simulink model "model_2"  (R2021b)
settings: Solver=ode23t  StartTime=0.0  StopTime=1e6
values from neighbouring files (symbols this model uses):
  Force_Vectors = [Force_Vectors;normal_vector]    [ellip_force_test.m]    (also in initial_sim.m = Force_Vectors'; initial_sim2.m = Force_Vectors'; multi_sim.m = Force_Vectors'; multi_sim2.m = Force_Vectors')
  max_f = 100000    [initial_sim.m]    (also in initial_sim2.m = 10)
  max_M_available = max_M_available*0.7    [initial_sim.m]    (also in initial_sim2.m; multi_sim.m; multi_sim2.m)
  Moment_Vectors = [Moment_Vectors;cross([x y z],normal_vector)]    [ellip_force_test.m]    (also in initial_sim.m = Moment_Vectors'; initial_sim2.m = Moment_Vectors'; multi_sim.m = Moment_Vectors'; multi_sim2.m = Moment_Vectors')
  N_sat = length(azimuths)    [ellip_force_test.m]    (also in initial_sim.m = 30; initial_sim2.m = 25; multi_sim.m = sim_data.N_sat; multi_sim2.m = sim_data.N_sat)
  params = 0    [Combo_OT.m]
undefined symbols (not defined in the file or in its folder): mp_0, mp_f
libraries: slpidlib x3, simulink x2, shared6dof x1
settings Model: Creator=Mehdi  LastModifiedBy=Mehdi

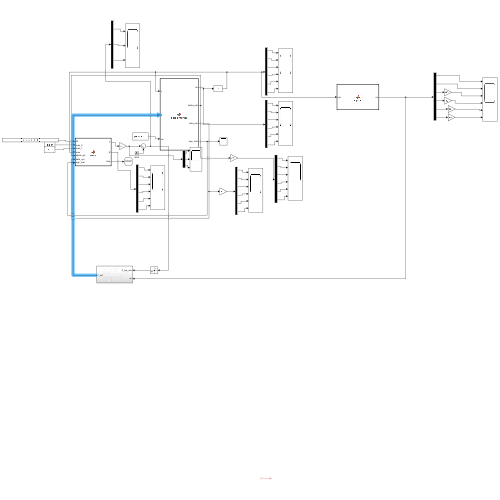
[thumbnail: Simulink's stored preview of the top-level diagram]
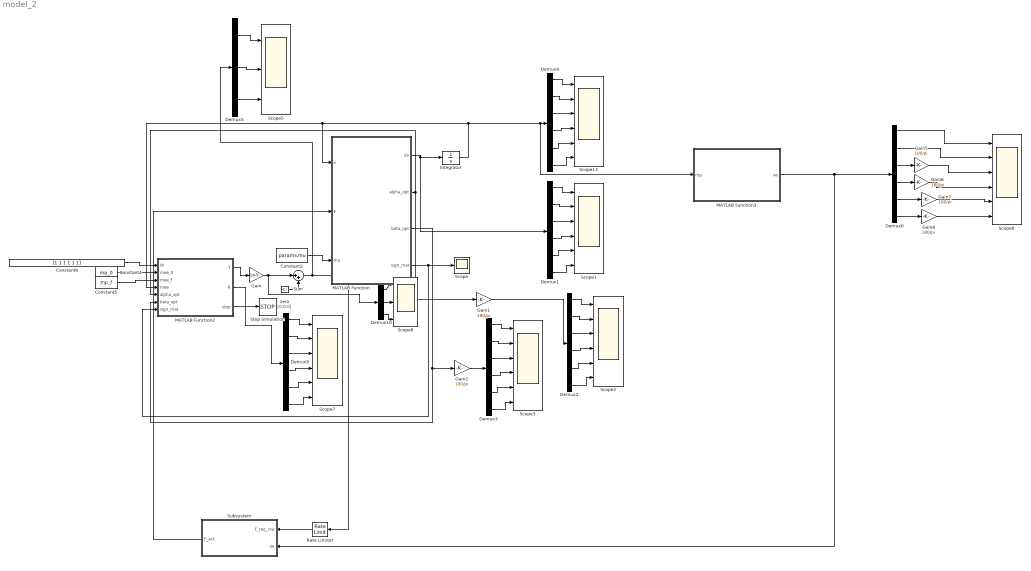
== system model_2 ==
  Constant2 : Constant  Value=params.mu
  Constant4 : Constant  Value=mp_0
  Constant5 : Constant  Value=mp_f
  Constant6 : Constant  Value=[1 1 1 1 1 1]
  Demux{1..3,6,8..9} (6 alike) : Demux  Outputs=6
  Demux10 : Demux  Outputs=3
  Demux5 : Demux  Outputs=3
  Gain : Gain  Gain=1e-5
  Gain{1..2,5..8} (6 alike) : Gain  Gain=180/pi
  Integrator : Integrator  InitialCondition=mp_0
  MATLAB Function : MATLAB Function  TreatAsAtomicUnit=on
  MATLAB Function2 : MATLAB Function  TreatAsAtomicUnit=on
  MATLAB Function3 : MATLAB Function  TreatAsAtomicUnit=on
  Rate Limiter : RateLimiter  RisingSlewLimit=1e-5  FallingSlewLimit=-1e-5  SampleTimeMode=inherited
  Scope : Scope
  Scope{1..3,6..7,13} (6 alike) : Scope  NumInputPorts=6
  Scope5 : Scope  NumInputPorts=3
  Scope8 : Scope  NumInputPorts=3
  Stop Simulation : Stop
  Subsystem : Subsystem
  Sum : Sum  Inputs=|++
  zero : Constant  Value=[0;0;0]
  wires:
  Integrator/1 -> MATLAB Function2/4(mee), MATLAB Function/1(x), MATLAB Function3/1(mp), Demux9/1
  Constant2/1 -> MATLAB Function/3(mu)
  Demux9/5 -> Scope13/5
  Demux9/1 -> Scope13/1
  Demux9/4 -> Scope13/4
  Demux9/3 -> Scope13/3
  Demux9/2 -> Scope13/2
  Demux9/6 -> Scope13/6
  Demux1/6 -> Scope1/6
  Demux1/2 -> Scope1/2
  Demux1/3 -> Scope1/3
  Demux1/4 -> Scope1/4
  Demux1/1 -> Scope1/1
  Demux1/5 -> Scope1/5
  Demux2/6 -> Scope2/6
  Demux2/2 -> Scope2/2
  Demux2/3 -> Scope2/3
  Demux2/4 -> Scope2/4
  Demux2/1 -> Scope2/1
  Demux2/5 -> Scope2/5
  MATLAB Function/2(alpha_opt) -> Gain1/1, MATLAB Function2/5(alpha_opt)
  MATLAB Function/3(beta_opt) -> MATLAB Function2/6(beta_opt), Gain2/1
  Demux3/5 -> Scope3/5
  Demux3/1 -> Scope3/1
  Demux3/4 -> Scope3/4
  Demux3/3 -> Scope3/3
  Demux3/2 -> Scope3/2
  Demux3/6 -> Scope3/6
  Constant4/1 -> MATLAB Function2/2(mee_0)
  Constant5/1 -> MATLAB Function2/3(mee_f)
  Constant6/1 -> MATLAB Function2/1(W)
  Demux5/3 -> Scope5/3
  Demux5/2 -> Scope5/2
  Demux5/1 -> Scope5/1
  MATLAB Function2/1(T) -> Gain/1
  zero/1 -> Sum/2
  Gain/1 -> Sum/1, Demux10/1
  MATLAB Function2/3(stop) -> Stop Simulation/1
  Demux6/6 -> Gain8/1
  Demux6/3 -> Gain5/1
  Demux6/4 -> Gain6/1
  Demux6/5 -> Gain7/1
  MATLAB Function3/1(oe) -> Subsystem/2(oe), Demux6/1
  Demux8/4 -> Scope7/4
  Demux8/3 -> Scope7/3
  Demux8/5 -> Scope7/5
  Demux8/2 -> Scope7/2
  Demux8/6 -> Scope7/6
  Demux8/1 -> Scope7/1
  MATLAB Function2/2(R) -> Demux8/1
  Gain1/1 -> Demux2/1
  MATLAB Function/1(dx) -> Demux1/1, Integrator/1
  Gain2/1 -> Demux3/1
  Demux6/1 -> Scope6/1
  Demux6/2 -> Scope6/2
  Gain5/1 -> Scope6/3
  Gain6/1 -> Scope6/4
  Gain7/1 -> Scope6/5
  Gain8/1 -> Scope6/6
  Demux10/2 -> Scope8/2
  Demux10/1 -> Scope8/1
  Demux10/3 -> Scope8/3
  ? -> ?
  Sum/1 -> Demux5/1, Rate Limiter/1
  Subsystem/1(F_act) -> MATLAB Function/2(F)
  Rate Limiter/1 -> Subsystem/1(F_req_rsw)
  MATLAB Function/4(sign_mat) -> MATLAB Function2/7(sign_mat), Scope/1

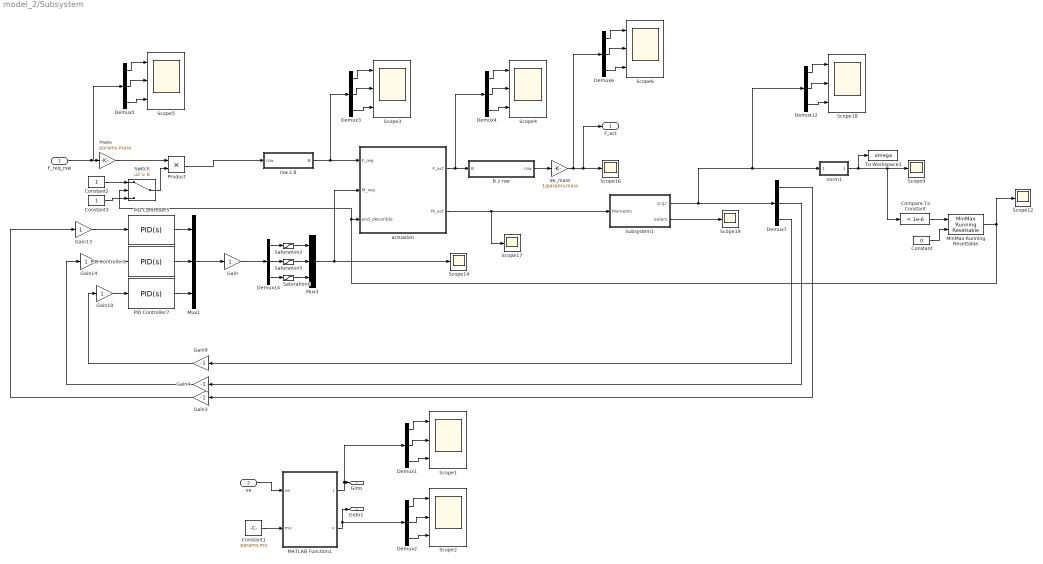
== system model_2/Subsystem ==
  F_req_rsw : Inport
  oe : Inport  Port=2
  B 2 rsw : Subsystem
  Compare To Constant : simulink/Logic and Bit Operations/Compare To Constant  relop=<  const=1e-6  OutDataTypeStr=boolean
  Constant : Constant  Value=0
  Constant1 : Constant  Value=params.mu
  Constant2 : Constant
  Constant3 : Constant
  Demux{1..7,12,14} (9 alike) : Demux  Outputs=3
  Gain{,10,13..14} (4 alike) : Gain
  Gain3 : Gain  Gain=-1
  Gain4 : Gain  Gain=-1
  Gain9 : Gain  Gain=-1
  MATLAB Function1 : MATLAB Function  TreatAsAtomicUnit=on
  MinMax Running Resettable : simulink/Math Operations/MinMax Running Resettable  Function=max  vinit=0.0
  Mux1 : Mux  Inputs=3
  Mux3 : Mux  Inputs=3
  PID Controller5 : slpidlib/PID Controller  Controller=PID  Form=Parallel  TimeDomain=Continuous-time  UseExternalTs=off  SampleTime=-1  IntegratorMethod=Forward Euler  FilterMethod=Forward Euler  ControllerParametersSource=internal  P=493.267124009933  I=0.0943532881280952  D=-103949.358808414  UseFilter=on  N=0.00172044274974478  TunerSelectOption=Transfer Function Based (PID Tuner App)  InitialConditionSource=internal  InitialConditionForIntegrator=0  InitialConditionForFilter=0  DifferentiatorICPrevScaledInput=0  ExternalReset=none  TrackingMode=off  Kt=1  LimitOutput=off  SatLimitsSource=internal  UpperSaturationLimit=inf  LowerSaturationLimit=-inf  LinearizeAsGain=on  AntiWindupMode=none  Kb=1  POutMin=[]  POutMax=[]  IOutMin=[]  IOutMax=[]  DOutMin=[]  DOutMax=[]  NOutMin=[]  NOutMax=[]  SumOutMin=[]  SumOutMax=[]  SaturationOutMin=[]  SaturationOutMax=[]  PParamMin=[]  PParamMax=[]  IParamMin=[]  IParamMax=[]  DParamMin=[]  DParamMax=[]  NParamMin=[]  NParamMax=[]  KbParamMin=[]  KbParamMax=[]  KtParamMin=[]  KtParamMax=[]  KbOutMin=[]  KbOutMax=[]  KtOutMin=[]  KtOutMax=[]  IntegratorOutMin=[]  IntegratorOutMax=[]  FilterOutMin=[]  FilterOutMax=[]  SumI1OutMin=[]  SumI1OutMax=[]  SumI2OutMin=[]  SumI2OutMax=[]  SumI3OutMin=[]  SumI3OutMax=[]  SumI4OutMin=[]  SumI4OutMax=[]  SumDOutMin=[]  SumDOutMax=[]  DifferentiatorOutMin=[]  DifferentiatorOutMax=[]  FilterDiffOutCoefMin=[]  FilterDiffOutCoefMax=[]  ReciprocalOutMin=[]  ReciprocalOutMax=[]  SumDenOutMin=[]  SumDenOutMax=[]  SumNumOutMin=[]  SumNumOutMax=[]  DivideOutMin=[]  DivideOutMax=[]  UdiffTsProdOutMin=[]  UdiffTsProdOutMax=[]  NTsProdOutMin=[]  NTsProdOutMax=[]  UintegralTsProdOutMin=[]  UintegralTsProdOutMax=[]  UngainTsProdOutMin=[]  UngainTsProdOutMax=[]  IntegratorContinuousStateAttributes=''  IntegratorStateMustResolveToSignalObject=off  IntegratorRTWStateStorageClass=Auto  FilterContinuousStateAttributes=''  FilterStateMustResolveToSignalObject=off  FilterRTWStateStorageClass=Auto  ParallelPVariant=InternalParameters  IdealPVariant=Disabled  IVariant=InternalParameters  DVariant=InternalParameters  IntegratorVariant=Continuous  SatVariant=Disabled  AWVariant=Passthrough  PCopyVariant=Disabled  TRVariant=Disabled  FdbkBlocksVariant=Forward  IdealPFdbkVariant=Disabled  SatFdbkVariant=Disabled  DerivativeFilterVariant=ContFilter  NVariant=InternalParameters  NCopyVariant=Disabled  FilterICVariant=InternalICsFilter  IntegratorICVariant=InternalICs  ExternalResetVariant=Disabled  TRSumVariant=Passthrough  SumFdbkVariant=Disabled  SumVariant=Sum_PID  TsampFilterVariant=InternalTs  TsampNgainVariant=Passthrough  TsampIntegralVariant=Passthrough  ExternalSaturationOutDataTypeStr=Inherit: Same as second input
  PID Controller6 : slpidlib/PID Controller  Controller=PID  Form=Parallel  TimeDomain=Continuous-time  UseExternalTs=off  SampleTime=-1  IntegratorMethod=Forward Euler  FilterMethod=Forward Euler  ControllerParametersSource=internal  P=493.267124009933  I=0.0943532881280952  D=-103949.358808414  UseFilter=on  N=0.00172044274974478  TunerSelectOption=Transfer Function Based (PID Tuner App)  InitialConditionSource=internal  InitialConditionForIntegrator=0  InitialConditionForFilter=0  DifferentiatorICPrevScaledInput=0  ExternalReset=none  TrackingMode=off  Kt=1  LimitOutput=off  SatLimitsSource=internal  UpperSaturationLimit=inf  LowerSaturationLimit=-inf  LinearizeAsGain=on  AntiWindupMode=none  Kb=1  POutMin=[]  POutMax=[]  IOutMin=[]  IOutMax=[]  DOutMin=[]  DOutMax=[]  NOutMin=[]  NOutMax=[]  SumOutMin=[]  SumOutMax=[]  SaturationOutMin=[]  SaturationOutMax=[]  PParamMin=[]  PParamMax=[]  IParamMin=[]  IParamMax=[]  DParamMin=[]  DParamMax=[]  NParamMin=[]  NParamMax=[]  KbParamMin=[]  KbParamMax=[]  KtParamMin=[]  KtParamMax=[]  KbOutMin=[]  KbOutMax=[]  KtOutMin=[]  KtOutMax=[]  IntegratorOutMin=[]  IntegratorOutMax=[]  FilterOutMin=[]  FilterOutMax=[]  SumI1OutMin=[]  SumI1OutMax=[]  SumI2OutMin=[]  SumI2OutMax=[]  SumI3OutMin=[]  SumI3OutMax=[]  SumI4OutMin=[]  SumI4OutMax=[]  SumDOutMin=[]  SumDOutMax=[]  DifferentiatorOutMin=[]  DifferentiatorOutMax=[]  FilterDiffOutCoefMin=[]  FilterDiffOutCoefMax=[]  ReciprocalOutMin=[]  ReciprocalOutMax=[]  SumDenOutMin=[]  SumDenOutMax=[]  SumNumOutMin=[]  SumNumOutMax=[]  DivideOutMin=[]  DivideOutMax=[]  UdiffTsProdOutMin=[]  UdiffTsProdOutMax=[]  NTsProdOutMin=[]  NTsProdOutMax=[]  UintegralTsProdOutMin=[]  UintegralTsProdOutMax=[]  UngainTsProdOutMin=[]  UngainTsProdOutMax=[]  IntegratorContinuousStateAttributes=''  IntegratorStateMustResolveToSignalObject=off  IntegratorRTWStateStorageClass=Auto  FilterContinuousStateAttributes=''  FilterStateMustResolveToSignalObject=off  FilterRTWStateStorageClass=Auto  ParallelPVariant=InternalParameters  IdealPVariant=Disabled  IVariant=InternalParameters  DVariant=InternalParameters  IntegratorVariant=Continuous  SatVariant=Disabled  AWVariant=Passthrough  PCopyVariant=Disabled  TRVariant=Disabled  FdbkBlocksVariant=Forward  IdealPFdbkVariant=Disabled  SatFdbkVariant=Disabled  DerivativeFilterVariant=ContFilter  NVariant=InternalParameters  NCopyVariant=Disabled  FilterICVariant=InternalICsFilter  IntegratorICVariant=InternalICs  ExternalResetVariant=Disabled  TRSumVariant=Passthrough  SumFdbkVariant=Disabled  SumVariant=Sum_PID  TsampFilterVariant=InternalTs  TsampNgainVariant=Passthrough  TsampIntegralVariant=Passthrough  ExternalSaturationOutDataTypeStr=Inherit: Same as second input
  PID Controller7 : slpidlib/PID Controller  Controller=PID  Form=Parallel  TimeDomain=Continuous-time  UseExternalTs=off  SampleTime=-1  IntegratorMethod=Forward Euler  FilterMethod=Forward Euler  ControllerParametersSource=internal  P=493.267124009933  I=0.0943532881280952  D=-103949.358808414  UseFilter=on  N=0.00172044274974478  TunerSelectOption=Transfer Function Based (PID Tuner App)  InitialConditionSource=internal  InitialConditionForIntegrator=0  InitialConditionForFilter=0  DifferentiatorICPrevScaledInput=0  ExternalReset=none  TrackingMode=off  Kt=1  LimitOutput=off  SatLimitsSource=internal  UpperSaturationLimit=inf  LowerSaturationLimit=-inf  LinearizeAsGain=on  AntiWindupMode=none  Kb=1  POutMin=[]  POutMax=[]  IOutMin=[]  IOutMax=[]  DOutMin=[]  DOutMax=[]  NOutMin=[]  NOutMax=[]  SumOutMin=[]  SumOutMax=[]  SaturationOutMin=[]  SaturationOutMax=[]  PParamMin=[]  PParamMax=[]  IParamMin=[]  IParamMax=[]  DParamMin=[]  DParamMax=[]  NParamMin=[]  NParamMax=[]  KbParamMin=[]  KbParamMax=[]  KtParamMin=[]  KtParamMax=[]  KbOutMin=[]  KbOutMax=[]  KtOutMin=[]  KtOutMax=[]  IntegratorOutMin=[]  IntegratorOutMax=[]  FilterOutMin=[]  FilterOutMax=[]  SumI1OutMin=[]  SumI1OutMax=[]  SumI2OutMin=[]  SumI2OutMax=[]  SumI3OutMin=[]  SumI3OutMax=[]  SumI4OutMin=[]  SumI4OutMax=[]  SumDOutMin=[]  SumDOutMax=[]  DifferentiatorOutMin=[]  DifferentiatorOutMax=[]  FilterDiffOutCoefMin=[]  FilterDiffOutCoefMax=[]  ReciprocalOutMin=[]  ReciprocalOutMax=[]  SumDenOutMin=[]  SumDenOutMax=[]  SumNumOutMin=[]  SumNumOutMax=[]  DivideOutMin=[]  DivideOutMax=[]  UdiffTsProdOutMin=[]  UdiffTsProdOutMax=[]  NTsProdOutMin=[]  NTsProdOutMax=[]  UintegralTsProdOutMin=[]  UintegralTsProdOutMax=[]  UngainTsProdOutMin=[]  UngainTsProdOutMax=[]  IntegratorContinuousStateAttributes=''  IntegratorStateMustResolveToSignalObject=off  IntegratorRTWStateStorageClass=Auto  FilterContinuousStateAttributes=''  FilterStateMustResolveToSignalObject=off  FilterRTWStateStorageClass=Auto  ParallelPVariant=InternalParameters  IdealPVariant=Disabled  IVariant=InternalParameters  DVariant=InternalParameters  IntegratorVariant=Continuous  SatVariant=Disabled  AWVariant=Passthrough  PCopyVariant=Disabled  TRVariant=Disabled  FdbkBlocksVariant=Forward  IdealPFdbkVariant=Disabled  SatFdbkVariant=Disabled  DerivativeFilterVariant=ContFilter  NVariant=InternalParameters  NCopyVariant=Disabled  FilterICVariant=InternalICsFilter  IntegratorICVariant=InternalICs  ExternalResetVariant=Disabled  TRSumVariant=Passthrough  SumFdbkVariant=Disabled  SumVariant=Sum_PID  TsampFilterVariant=InternalTs  TsampNgainVariant=Passthrough  TsampIntegralVariant=Passthrough  ExternalSaturationOutDataTypeStr=Inherit: Same as second input
  Product : Product
  Saturation2 : Saturate  UpperLimit=max_M_available(1,1)  LowerLimit=max_M_available(1,2)
  Saturation5 : Saturate  UpperLimit=max_M_available(2,1)  LowerLimit=max_M_available(2,2)
  Saturation6 : Saturate  UpperLimit=max_M_available(3,1)  LowerLimit=max_M_available(3,2)
  Scope{1..6,18} (7 alike) : Scope  NumInputPorts=3
  Scope{9,12,14,16..17,19} (6 alike) : Scope
  Subsystem1 : Subsystem
  Switch : Switch  Criteria=u2 > Threshold
  To Workspace1 : ToWorkspace  VariableName=omega  SaveFormat=Timeseries  SampleTime=-1
      settings: MaxDataPoints=1
  actuation : Subsystem
  de_mass : Gain  Gain=1/params.mass
  mass : Gain  Gain=params.mass
  norm1 : Subsystem
  rsw 2 B : Subsystem
  F_act : Outport
  tag scope: r=global, v=global
  wires:
  PID Controller5/1 -> Mux1/1
  norm1/1(Out1) -> To Workspace1/1, Scope9/1, Compare To Constant/1
  Gain9/1 -> Gain10/1
  Gain10/1 -> PID Controller7/1
  Gain3/1 -> Gain13/1
  actuation/2(M_act) -> Subsystem1/1(Moments), Scope17/1
  B 2 rsw/1(rsw) -> de_mass/1
  Subsystem1/1(p,q,r) -> Demux12/1, norm1/1(p,q,r), Demux7/1
  Mux1/1 -> Gain/1
  Demux7/2 -> Gain4/1
  Saturation5/1 -> Mux3/2
  rsw 2 B/1(B) -> Demux3/1, actuation/1(F_req)
  Gain4/1 -> Gain14/1
  Demux7/3 -> Gain9/1
  Demux14/3 -> Saturation6/1
  Demux12/2 -> Scope18/2
  Saturation2/1 -> Mux3/1
  Demux12/1 -> Scope18/1
  actuation/1(F_act) -> Demux4/1, B 2 rsw/1(B)
  Mux3/1 -> actuation/2(M_req), Scope14/1
  Subsystem1/2(eulers) -> Scope19/1
  PID Controller7/1 -> Mux1/3
  Demux14/1 -> Saturation2/1
  Demux12/3 -> Scope18/3
  Demux14/2 -> Saturation5/1
  MinMax Running Resettable/1 -> Scope12/1, actuation/3(end_detumble), Switch/2
  Gain13/1 -> PID Controller5/1
  Compare To Constant/1 -> MinMax Running Resettable/1
  Gain14/1 -> PID Controller6/1
  Constant/1 -> MinMax Running Resettable/2
  Demux7/1 -> Gain3/1
  PID Controller6/1 -> Mux1/2
  Saturation6/1 -> Mux3/3
  MATLAB Function1/1(r) -> Demux1/1, [r]
  MATLAB Function1/2(v) -> Demux2/1, [v]
  Constant1/1 -> MATLAB Function1/2(mu)
  oe/1 -> MATLAB Function1/1(oe)
  Demux1/3 -> Scope1/3
  Demux1/1 -> Scope1/1
  Demux1/2 -> Scope1/2
  Demux2/3 -> Scope2/3
  Demux2/2 -> Scope2/2
  Demux2/1 -> Scope2/1
  Demux3/3 -> Scope3/3
  Demux3/1 -> Scope3/1
  Demux3/2 -> Scope3/2
  Demux4/2 -> Scope4/2
  Demux4/1 -> Scope4/1
  Demux4/3 -> Scope4/3
  F_req_rsw/1 -> Demux5/1, mass/1
  Demux5/2 -> Scope5/2
  Demux5/1 -> Scope5/1
  Demux5/3 -> Scope5/3
  Demux6/3 -> Scope6/3
  Demux6/1 -> Scope6/1
  Demux6/2 -> Scope6/2
  de_mass/1 -> Demux6/1, F_act/1, Scope16/1
  mass/1 -> Product/1
  Product/1 -> rsw 2 B/1(rsw)
  Switch/1 -> Product/2
  Constant2/1 -> Switch/1
  Constant3/1 -> Switch/3
  Gain/1 -> Demux14/1

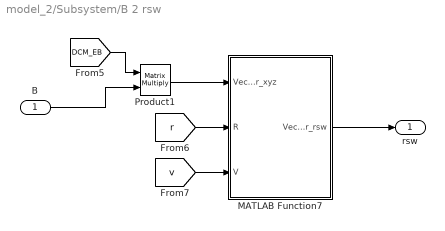
== system model_2/Subsystem/B 2 rsw ==
  B : Inport
  MATLAB Function7 : MATLAB Function  TreatAsAtomicUnit=on
  Product1 : Product  Multiplication=Matrix(*)
  rsw : Outport
  wires:
  Product1/1 -> MATLAB Function7/1(Vector_xyz)
  [v] -> MATLAB Function7/3(V)
  [DCM_EB] -> Product1/1
  [r] -> MATLAB Function7/2(R)
  B/1 -> Product1/2
  MATLAB Function7/1(Vector_rsw) -> rsw/1

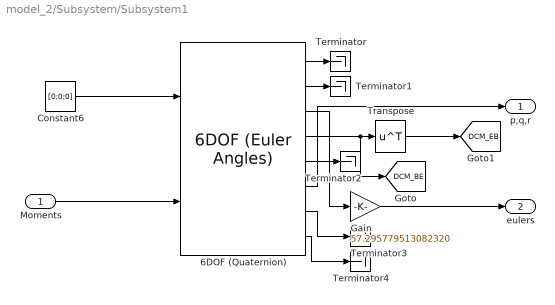
== system model_2/Subsystem/Subsystem1 ==
  Moments : Inport
  6DOF (Quaternion) : shared6dof/6DOF (Euler Angles)  units=Metric (MKS)  mtype=Fixed  rep=Quaternion  xme_0=[0 0 0]  Vm_0=[0 0 0]  eul_0=eul_0  pm_0=pqr_0  mass_0=1.0  mass_e=0.5  mass_f=2.0  inertia=params.Inertia  inertia_e=eye(3)  inertia_f=2*eye(3)  k_quat=1.0  vre_flag=on  abi_flag=off  aMode=0  xme_statename=''  Vm_statename=''  eul_statename=''  quat_statename=''  pm_statename=''  mass_statename=''
      settings: SourceProductBaseCode=AE,PW,DR,MT,UV,VE
  Constant6 : Constant  Value=[0;0;0]
  Gain : Gain  Gain=57.295779513082320
  Terminator{,1..4} (5 alike) : Terminator
  Transpose : Math  Operator=transpose  SaturateOnIntegerOverflow=on
  p,q,r : Outport
  eulers : Outport  Port=2
  tag scope: DCM_BE=global, DCM_EB=global
  wires:
  6DOF (Quaternion)/7 -> Terminator3/1
  Constant6/1 -> 6DOF (Quaternion)/1
  6DOF (Quaternion)/3 -> Gain/1
  6DOF (Quaternion)/1 -> Terminator/1
  6DOF (Quaternion)/6 -> p,q,r/1
  6DOF (Quaternion)/5 -> Terminator2/1
  6DOF (Quaternion)/2 -> Terminator1/1
  Gain/1 -> eulers/1
  6DOF (Quaternion)/4 -> [DCM_BE], Transpose/1
  6DOF (Quaternion)/8 -> Terminator4/1
  Moments/1 -> 6DOF (Quaternion)/2
  Transpose/1 -> [DCM_EB]

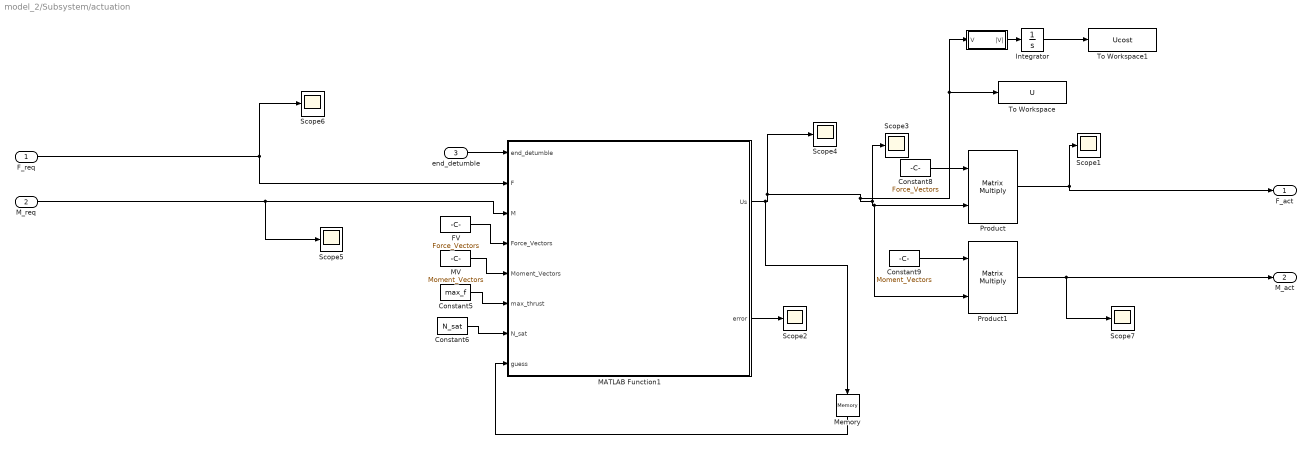
== system model_2/Subsystem/actuation ==
  F_req : Inport
  M_req : Inport  Port=2
  end_detumble : Inport  Port=3
  " " : Subsystem
  Constant5 : Constant  Value=max_f
  Constant6 : Constant  Value=N_sat
  Constant8 : Constant  Value=Force_Vectors
  Constant9 : Constant  Value=Moment_Vectors
  FV : Constant  Value=Force_Vectors
  Integrator : Integrator
  MATLAB Function1 : MATLAB Function  TreatAsAtomicUnit=on
  MV : Constant  Value=Moment_Vectors
  Memory : Memory  InitialCondition=zeros(N_sat,1)
  Product : Product  Multiplication=Matrix(*)
  Product1 : Product  Multiplication=Matrix(*)
  Scope{1..7} (7 alike) : Scope
  To Workspace : ToWorkspace  VariableName=U  SaveFormat=Timeseries  SampleTime=-1
  To Workspace1 : ToWorkspace  VariableName=Ucost  SaveFormat=Timeseries  SampleTime=-1
      settings: MaxDataPoints=1
  F_act : Outport
  M_act : Outport  Port=2
  wires:
  Constant6/1 -> MATLAB Function1/7(N_sat)
  Constant9/1 -> Product1/1
  Memory/1 -> MATLAB Function1/8(guess)
  MATLAB Function1/2(error) -> Scope2/1
  FV/1 -> MATLAB Function1/4(Force_Vectors)
  MV/1 -> MATLAB Function1/5(Moment_Vectors)
  Product1/1 -> Scope7/1, M_act/1
  Constant8/1 -> Product/1
  Constant5/1 -> MATLAB Function1/6(max_thrust)
  F_req/1 -> MATLAB Function1/2(F), Scope6/1
  Product/1 -> F_act/1, Scope1/1
  end_detumble/1 -> MATLAB Function1/1(end_detumble)
  MATLAB Function1/1(Us) -> Scope4/1, Product/2, Product1/2, Scope3/1, " "/1(V), To Workspace/1, Memory/1
  " "/1(|V|) -> Integrator/1
  Integrator/1 -> To Workspace1/1
  M_req/1 -> MATLAB Function1/3(M), Scope5/1

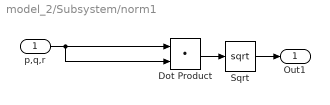
== system model_2/Subsystem/norm1 ==
  p,q,r : Inport
  Dot Product : DotProduct  InputSameDT=on  OutDataTypeStr=Inherit: Inherit via internal rule
  Sqrt : Sqrt  OutputSignalType=real  SaturateOnIntegerOverflow=on
  Out1 : Outport
  wires:
  Dot Product/1 -> Sqrt/1
  p,q,r/1 -> Dot Product/1, Dot Product/2
  Sqrt/1 -> Out1/1

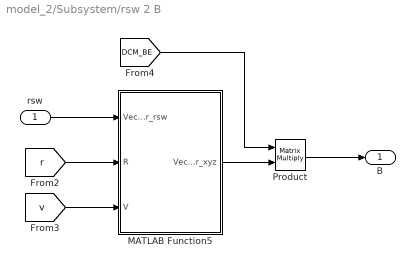
== system model_2/Subsystem/rsw 2 B ==
  rsw : Inport
  MATLAB Function5 : MATLAB Function  TreatAsAtomicUnit=on
  Product : Product  Multiplication=Matrix(*)
  B : Outport
  wires:
  [DCM_BE] -> Product/1
  rsw/1 -> MATLAB Function5/1(Vector_rsw)
  MATLAB Function5/1(Vector_xyz) -> Product/2
  [v] -> MATLAB Function5/3(V)
  [r] -> MATLAB Function5/2(R)
  Product/1 -> B/1

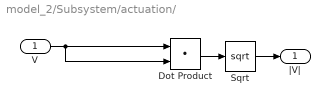
== system model_2/Subsystem/actuation/  ==
  V : Inport
  Dot Product : DotProduct  InputSameDT=on  OutDataTypeStr=Inherit: Inherit via internal rule
  Sqrt : Sqrt  OutputSignalType=real  SaturateOnIntegerOverflow=on
  |V| : Outport
  wires:
  Dot Product/1 -> Sqrt/1
  V/1 -> Dot Product/1, Dot Product/2
  Sqrt/1 -> |V|/1

== matlab function model_2/Subsystem/B 2 rsw/MATLAB Function7 ==
  data: Vector_xyz input; R input; Vector_rsw output; V input
function Vector_rsw=xyz2rsw(Vector_xyz,R,V)

Vector_rsw=zeros(3,1);

e_r=R/norm(R);
h=cross(R,V);
e_w=h/norm(h);
e_s=cross(e_w,e_r);


Vector_rsw(1)=dot(Vector_xyz,e_r);
Vector_rsw(2)=dot(Vector_xyz,e_s);
Vector_rsw(3)=dot(Vector_xyz,e_w);

end

== matlab function model_2/Subsystem/actuation/MATLAB Function1 ==
  data: end_detumble input; F input size=3; Us output; M input size=3; Force_Vectors input; Moment_Vectors input; error output; max_thrust input; N_sat input size=1; guess input
function [Us,error] = cotrol_allocation(end_detumble,F,M,Force_Vectors,Moment_Vectors,max_thrust,N_sat,guess)


maxIter=10;

% Us=zeros(N_sat,1);
% Uss=zeros(N_sat,1);
if end_detumble==0
    %     b=[F(1);F(2);F(3);0;0;0];
    b=[F(1);F(2);F(3);M(1);M(2);M(3)];
else
    b=[F(1);F(2);F(3);0;0;0];
    %     b=[0;0;0;M(1);M(2);M(3)];
end
C=[Force_Vectors;Moment_Vectors];

options = optimoptions('lsqnonlin','Algorithm','levenberg-marquardt','MaxIterations',maxIter);
LB=zeros(N_sat,1);
UB=max_thrust*ones(N_sat,1);
% x0=zeros(N_sat,1);
x0=guess;

% C*x0-b

fun=@(x)(C*x-b);



[Uss,error]=lsqnonlin(fun,x0,LB,UB,options);


if error<1e-6
    
    
    Us=Uss(1:30,1);
    
else
    
    Us=zeros(30,1);
    
end

%
% F_out=Force_Vectors*Us;
% M_out=Moment_Vectors*Us;



% Us=C*x0-b;


% for i=1:N_sat
%     Us(i)=U1(i);
% end

% error=0;


end

== matlab function model_2/MATLAB Function ==
  data: x input; F input; dx output; mu input; alpha_opt output; beta_opt output; sign_mat output
function [dx,alpha_opt,beta_opt,sign_mat] = path_dynamics(x,F,mu)

% a
% ep1=e*sin(omega+OMEGA);
% ep2=e*cos(omega+OMEGA);
% zig1=tan(inc/2)*sin(OMEGA);
% zig2=tan(inc/2)*cos(OMEGA);
% lambda=theta+omega+OMEGA;


a=x(1);
ep1=x(2);
ep2=x(3);
zig1=x(4);
zig2=x(5);
lambda=x(6);

slam=sin(lambda);
clam=cos(lambda);
L=a*(1-ep1^2-ep2^2);
h=sqrt(mu*L);
r=L/(1+ep1*slam+ep2*clam);

%%% to be optimized!

a_dot=2*a^2/h*dot([ep2*slam-ep1*clam L/r 0],F);
ep1_dot=r/h*dot([-L/r*clam ep1+(1+L/r)*slam -ep2*(zig1*clam-zig2*slam)],F);
ep2_dot=r/h*dot([L/r*slam ep2+(1+L/r)*clam ep1*(zig1*clam-zig2*slam)],F);
zig1_dot=r/(2*h)*dot([0 0 (1+zig1^2+zig2^2)*slam],F);
zig2_dot=r/(2*h)*dot([0 0 (1+zig1^2+zig2^2)*clam],F);
lambda_dot=h/r^2+r/h*dot([0 0 zig2*slam-zig1*clam],F);

% dx=zeros(6,1);

dx=[a_dot;ep1_dot;ep2_dot;zig1_dot;zig2_dot;lambda_dot];


% sign_mat=sign([ep2*slam-ep1*clam L/r 0;-L/r*clam ep1+(1+L/r)*slam -ep2*(zig1*clam-zig2*slam);L/r*slam ep2+(1+L/r)*clam ep1*(zig1*clam-zig2*slam);0 0 (1+zig1^2+zig2^2)*slam;0 0 (1+zig1^2+zig2^2)*clam;0 0 zig2*slam-zig1*clam]);
sign_mat=sign([ep2*slam-ep1*clam 1 0;-clam ep1+(1+L/r)*slam -ep2*(zig1*clam-zig2*slam);slam ep2+(1+L/r)*clam ep1*(zig1*clam-zig2*slam);0 0 slam;0 0 clam;0 0 zig2*slam-zig1*clam]);



alpha_opt=zeros(6,1);
beta_opt=zeros(6,1);



alpha_opt(1)=atan(r/L*(ep2*slam-ep1*clam));
alpha_opt(2)=atan(-L*clam/(r*ep1+(r+L)*slam));
alpha_opt(3)=atan(L*slam/(r*ep2+(r+L)*clam));


beta_opt(2)=atan(r*ep2*(zig1*clam-zig2*slam)/(L*clam*sin(alpha_opt(2))-(r*ep1+(r+L)*slam)*cos(alpha_opt(2))));
beta_opt(3)=atan(r*ep1*(zig1*clam-zig2*slam)/(L*slam*sin(alpha_opt(3))-(r*ep2+(r+L)*clam)*cos(alpha_opt(3))));

beta_opt(4)=sign(slam)*pi/2;
beta_opt(5)=sign(clam)*pi/2;

beta_opt(6)=sign(zig2*slam-zig1*clam)*pi/2;


% e=sqrt(ep1^2+ep2^2);
% inc=2*atan(sqrt(zig1^2+zig2^2));
% OMEGA=atan(zig1/zig2);
% omega=atan(ep1/ep2)-OMEGA;
% theta=lambda-atan(ep1/ep2);








end

== matlab function model_2/MATLAB Function2 ==
  data: W input; mee_0 input; mee_f input; mee input; alpha_opt input; beta_opt input; T output; R output; stop output; sign_mat input
function [T,R,stop]  = Guider(W,mee_0,mee_f,mee,alpha_opt,beta_opt,sign_mat)


stop=0;

R=zeros(6,1);
ss=ones(6,1);

T=[0;0;0];

for i=1:6
    
    if abs(mee_f(i)-mee_0(i))>1e-5 && abs(mee_f(i)-mee(i))>1e-5
        
        R(i)=(mee(i)-mee_f(i))/(mee_f(i)-mee_0(i));
        
        if  abs(R(i))>5
            R(i)=5;
        end
        if  abs(R(i))<-5
            R(i)=-5;
        end
        
    end
end

if norm(R)<1e-2
    stop=1;
end





% % % ss(1)=sign(mee_f(1)-mee(1));  %% sign ok
% % % ss(2)=-sign(mee_f(2)-mee(2));  %% sign ok
% % % ss(3)=-sign(mee_f(3)-mee(3));
% % % ss(4)=sign(mee_f(4)-mee(4));
% % % ss(5)=sign(mee_f(5)-mee(5));
% % % ss(6)=sign(mee_f(6)-mee(6));

% ss=R_dot;

% ang1=rem(x(6)+2*pi,2*pi);
% if ang1>pi
%     ss(2)=-ss(2);
% alpha_opt(2)=2*pi-alpha_opt(2);
% end

% n=0;

for i=1:6
%     n=n+1;
    %     ss=1;
    %     ang1=rem(x(6)+2*pi,2*pi);
    %     if ang1<pi
    %         alpha_opt(i)=-alpha_opt(i);
    % ss=-1;
    %     end
    
    %         ss=sign(x(i)-mp_f(i));
    %     ss=1;
    %
    % ss=-1;

    if sign_mat(i,1)==-1
        alpha_opt(i)=-abs(alpha_opt(i));
    else
        alpha_opt(i)=abs(alpha_opt(i));
    end

    if sign_mat(i,3)==-1
        beta_opt(i)=-abs(beta_opt(i));
    else
        beta_opt(i)=abs(beta_opt(i));
    end


    T=T+ss(i)*W(i)*R(i)*([sin(alpha_opt(i))*cos(beta_opt(i));cos(alpha_opt(i))*cos(beta_opt(i));sin(beta_opt(i))]);
% T=T+ss(n)*W(n)*R(i)*([sin(alpha_opt(i))*cos(0);cos(alpha_opt(i))*cos(0);sin(beta_opt(i))]);
    %
end

% for i=1:6
%     n=n+1;
    %     ss=1;
    %     ang1=rem(x(6)+2*pi,2*pi);
    %     if ang1<pi
    %         alpha_opt(i)=-alpha_opt(i);
    % ss=-1;
    %     end
    
    %         ss=sign(x(i)-mp_f(i));
    %     ss=1;
    %
    % ss=-1;
%     T=T+ss(i)*W(i)*R(i)*([sin(alpha_opt(i))*cos(beta_opt(i));cos(alpha_opt(i))*cos(beta_opt(i));sin(beta_opt(i))]);
% T=T+ss(i)*W(n)*R(i)*([sin(0)*cos(beta_opt(i));cos(0)*cos(beta_opt(i));sin(beta_opt(i))]);
    %
% end


if norm(T)>0
    
    T=T./norm(T);
    
else
    T=[0;0;0];
end

end

== matlab function model_2/MATLAB Function3 ==
  data: mp input; oe output
function oe=mp2oe(mp)


a=mp(1);
ep1=mp(2);
ep2=mp(3);
zig1=mp(4);
zig2=mp(5);
lambda=mp(6);


% % ep1=e*sin(omega+OMEGA);
% % ep2=e*cos(omega+OMEGA);
% % zig1=tan(inc/2)*sin(OMEGA);
% % zig2=tan(inc/2)*cos(OMEGA);
% % lambda=theta+omega+OMEGA;
% %
% % mp=[a;ep1;ep2;zig1;zig2;lambda];

%%% to be optimized
e=sqrt(ep1^2+ep2^2);
inc=2*atan(sqrt(zig1^2+zig2^2));

if inc==0
    OMEGA=0;
else
    tan1=tan(inc/2);
    OMEGA=atan3(zig1/tan1,zig2/tan1);
end


% if sign(zig2)*sign(cos(OMEGA))<0 || sign(zig1)*sign(sin(OMEGA))<0
%     inc=-inc;
% end


if OMEGA>pi
    OMEGA=OMEGA-2*pi;
end

% inc=inc*(sign(zig2)*sign(cos(OMEGA)));

if e==0
    omega=0;
else
    omega=atan3(ep1/e,ep2/e)-OMEGA;
end

if omega>2*pi
    omega=omega-2*pi;
    
end


theta=lambda-omega-OMEGA;
if theta<0
    theta=theta+2*pi;
end

if theta>2*pi
    theta=rem(theta,2*pi);
end

oe=[a;e;inc;omega;OMEGA;theta];


end

== matlab function model_2/Subsystem/MATLAB Function1 ==
  data: oe input; r output; mu input; v output
function [r, v] = oe2rv(oe,mu)


% convert classical orbital elements to eci state vector

% input

%  mu     = gravitational constant (km**3/sec**2)
%  oev(1) = semimajor axis (kilometers)
%  oev(2) = orbital eccentricity (non-dimensional)
%           (0 <= eccentricity < 1)
%  oev(3) = orbital inclination (radians)
%           (0 <= inclination <= pi)
%  oev(4) = argument of perigee (radians)
%           (0 <= argument of perigee <= 2 pi)
%  oev(5) = right ascension of ascending node (radians)
%           (0 <= raan <= 2 pi)
%  oev(6) = true anomaly (radians)
%           (0 <= true anomaly <= 2 pi)

% output

%  r = eci position vector (kilometers)
%  v = eci velocity vector (kilometers/second)

% Orbital Mechanics with MATLAB

%%%%%%%%%%%%%%%%%%%%%%%%%%%%%%%

r = zeros(3, 1);
v = zeros(3, 1);

% unload orbital elements array
   
sma = oe(1);
ecc = oe(2);
inc = oe(3);
argper = oe(4);
raan = oe(5);
tanom = oe(6);

slr = sma * (1 - ecc * ecc);

rm = slr / (1 + ecc * cos(tanom));
   
arglat = argper + tanom;

sarglat = sin(arglat);
carglat = cos(arglat);
   
c4 = sqrt(mu / slr);
c5 = ecc * cos(argper) + carglat;
c6 = ecc * sin(argper) + sarglat;

sinc = sin(inc);
cinc = cos(inc);

sraan = sin(raan);
craan = cos(raan);

% position vector

r(1) = rm * (craan * carglat - sraan * cinc * sarglat);
r(2) = rm * (sraan * carglat + cinc * sarglat * craan);
r(3) = rm * sinc * sarglat;

% velocity vector

v(1) = -c4 * (craan * c6 + sraan * cinc * c5);
v(2) = -c4 * (sraan * c6 - craan * cinc * c5);
v(3) = c4 * c5 * sinc;
   
end

== matlab function model_2/Subsystem/rsw 2 B/MATLAB Function5 ==
  data: Vector_rsw input; R input; Vector_xyz output; V input
function Vector_xyz=rsw2xyz(Vector_rsw,R,V)



e_r=R/norm(R);
h=cross(R,V);
e_w=h/norm(h);
e_s=cross(e_w,e_r);


Vector_xyz=Vector_rsw(1)*e_r+Vector_rsw(2)*e_s+Vector_rsw(3)*e_w;


end
